simulink model "rfsoc_sdfec_model"  (R2020b)
settings: Solver=VariableStepAuto  StartTime=0.0  StopTime=T  RelTol=1e-3
values from neighbouring files (symbols this model uses):
  aximm_bit_count_reset = 0    [setup.m]
  aximm_bits = n_blocks * k    (= 80)    [setup.m]
  aximm_ctrl_word_dec = 0    [setup.m]
  aximm_ctrl_word_enc = 999    [setup.m]
  aximm_enable = 1    [setup.m]
  aximm_length = k * n_blocks    (= 80)    [setup.m]
  aximm_length_dec = n    (= 160)    [setup.m]
  aximm_length_enc = k/8    (= 10)    [setup.m]
  aximm_llr_scale = (1/noise_var) * llr_scale * 2    (= 200)    [setup.m]
  aximm_noise_std = sqrt(noise_var/2)    [setup.m]
  aximm_reset = 0    [setup.m]
  d = sqrt(-2*log([0:1/4095:1]))    [setup.m]
  fs = 100e6    (= 100000000)    [setup.m]
  generator_polynomial = '''z^13 + z^12 + z^11 + z^8 + 1'''    [setup.m]
libraries: hdlsllib x52, commseqgen3 x28, commblkcod2 x2, simulink x2
(part 2 of 2)

== system rfsoc_sdfec_model/Soft Demodulation/symmetric saturation1 ==
  soft_bits : Inport
  Bit Concat : hdlsllib/Logic and Bit Operations/Bit Concat  numInputs=3
  Bit Slice : hdlsllib/Logic and Bit Operations/Bit Slice  lidx=5  ridx=5
      settings: SourceProductBaseCode=SL
  Constant : Constant  Value=7.75  OutDataTypeStr=fixdt(1,6,2)  SampleTime=-1
  Constant2 : Constant  Value=-7.75  OutDataTypeStr=fixdt(1,6,2)  SampleTime=-1
  GreaterThan : RelationalOperator  Operator=>  OutDataTypeStr=boolean  RndMeth=Simplest
  GreaterThan1 : RelationalOperator  Operator=<  OutDataTypeStr=boolean  RndMeth=Simplest
  Multiport Switch : MultiPortSwitch  DataPortOrder=Zero-based contiguous  Inputs=2  zeroidx=on
  Multiport Switch1 : MultiPortSwitch  DataPortOrder=Zero-based contiguous  Inputs=2  zeroidx=on
  u : Outport
  wires:
  Constant2/1 -> Multiport Switch1/3, GreaterThan1/2
  Constant/1 -> Multiport Switch/3, GreaterThan/2
  Multiport Switch/1 -> Multiport Switch1/2
  GreaterThan1/1 -> Multiport Switch1/1
  GreaterThan/1 -> Multiport Switch/1
  soft_bits/1 -> GreaterThan1/1, Multiport Switch/2, GreaterThan/1
  Bit Concat/1 -> u/1
  Multiport Switch1/1 -> Bit Slice/1, Bit Concat/3
  Bit Slice/1 -> Bit Concat/2, Bit Concat/1

== system rfsoc_sdfec_model/Soft Demodulation/symmetric saturation2 ==
  soft_bits : Inport
  Bit Concat : hdlsllib/Logic and Bit Operations/Bit Concat  numInputs=3
  Bit Slice : hdlsllib/Logic and Bit Operations/Bit Slice  lidx=5  ridx=5
      settings: SourceProductBaseCode=SL
  Constant : Constant  Value=7.75  OutDataTypeStr=fixdt(1,6,2)  SampleTime=-1
  Constant2 : Constant  Value=-7.75  OutDataTypeStr=fixdt(1,6,2)  SampleTime=-1
  GreaterThan : RelationalOperator  Operator=>  OutDataTypeStr=boolean  RndMeth=Simplest
  GreaterThan1 : RelationalOperator  Operator=<  OutDataTypeStr=boolean  RndMeth=Simplest
  Multiport Switch : MultiPortSwitch  DataPortOrder=Zero-based contiguous  Inputs=2  zeroidx=on
  Multiport Switch1 : MultiPortSwitch  DataPortOrder=Zero-based contiguous  Inputs=2  zeroidx=on
  u : Outport
  wires:
  Bit Slice/1 -> Bit Concat/1, Bit Concat/2
  Multiport Switch1/1 -> Bit Concat/3, Bit Slice/1
  Bit Concat/1 -> u/1
  soft_bits/1 -> GreaterThan/1, Multiport Switch/2, GreaterThan1/1
  GreaterThan/1 -> Multiport Switch/1
  GreaterThan1/1 -> Multiport Switch1/1
  Multiport Switch/1 -> Multiport Switch1/2
  Constant/1 -> GreaterThan/2, Multiport Switch/3
  Constant2/1 -> GreaterThan1/2, Multiport Switch1/3

== system rfsoc_sdfec_model/Soft Demodulation/symmetric saturation3 ==
  soft_bits : Inport
  Bit Concat : hdlsllib/Logic and Bit Operations/Bit Concat  numInputs=3
  Bit Slice : hdlsllib/Logic and Bit Operations/Bit Slice  lidx=5  ridx=5
      settings: SourceProductBaseCode=SL
  Constant : Constant  Value=7.75  OutDataTypeStr=fixdt(1,6,2)  SampleTime=-1
  Constant2 : Constant  Value=-7.75  OutDataTypeStr=fixdt(1,6,2)  SampleTime=-1
  GreaterThan : RelationalOperator  Operator=>  OutDataTypeStr=boolean  RndMeth=Simplest
  GreaterThan1 : RelationalOperator  Operator=<  OutDataTypeStr=boolean  RndMeth=Simplest
  Multiport Switch : MultiPortSwitch  DataPortOrder=Zero-based contiguous  Inputs=2  zeroidx=on
  Multiport Switch1 : MultiPortSwitch  DataPortOrder=Zero-based contiguous  Inputs=2  zeroidx=on
  u : Outport
  wires:
  Constant2/1 -> Multiport Switch1/3, GreaterThan1/2
  Constant/1 -> Multiport Switch/3, GreaterThan/2
  Multiport Switch/1 -> Multiport Switch1/2
  GreaterThan1/1 -> Multiport Switch1/1
  GreaterThan/1 -> Multiport Switch/1
  soft_bits/1 -> GreaterThan1/1, Multiport Switch/2, GreaterThan/1
  Bit Concat/1 -> u/1
  Multiport Switch1/1 -> Bit Slice/1, Bit Concat/3
  Bit Slice/1 -> Bit Concat/2, Bit Concat/1

== system rfsoc_sdfec_model/AWGN Channel/AWGN Generator/Random Number Generator ==
  reset : Inport
  enable : EnablePort
  bit0 : commseqgen3/PN Sequence Generator  poly='z^13 + z^12 + z^11 + z^8 + 1'  ini_sta=[ 1 1 1 1 1 1 0 0 1 0 0 0 0]  outBitMaskSource=Dialog parameter  shift=0  outVarSiz=off  maxOutSizeMode=Dialog parameter  maxOutSize=[10 1]  Ts=-1  sampPerFrame=1  reset=on  bitPackedOutputs=off  outDataType=boolean  numPackedBits=8  bitPackDataSigned=off  bitPackedOutDType=double
  bit1 : commseqgen3/PN Sequence Generator  poly='z^13 + z^12 + z^11 + z^8 + 1'  ini_sta=[ 1 1 1 1 1 1 0 0 0 1 0 1 1]  outBitMaskSource=Dialog parameter  shift=0  outVarSiz=off  maxOutSizeMode=Dialog parameter  maxOutSize=[10 1]  Ts=-1  sampPerFrame=1  reset=on  bitPackedOutputs=off  outDataType=boolean  numPackedBits=8  bitPackDataSigned=off  bitPackedOutDType=double
  bit2 : commseqgen3/PN Sequence Generator  poly='z^13 + z^12 + z^11 + z^8 + 1'  ini_sta=[ 0 1 1 1 0 1 0 0 1 1 0 0 0]  outBitMaskSource=Dialog parameter  shift=0  outVarSiz=off  maxOutSizeMode=Dialog parameter  maxOutSize=[10 1]  Ts=-1  sampPerFrame=1  reset=on  bitPackedOutputs=off  outDataType=boolean  numPackedBits=8  bitPackDataSigned=off  bitPackedOutDType=double
  bit3 : commseqgen3/PN Sequence Generator  poly='z^13 + z^12 + z^11 + z^8 + 1'  ini_sta=[ 0 1 0 1 1 0 0 1 0 0 0 1 1]  outBitMaskSource=Dialog parameter  shift=0  outVarSiz=off  maxOutSizeMode=Dialog parameter  maxOutSize=[10 1]  Ts=-1  sampPerFrame=1  reset=on  bitPackedOutputs=off  outDataType=boolean  numPackedBits=8  bitPackDataSigned=off  bitPackedOutDType=double
  bit4 : commseqgen3/PN Sequence Generator  poly='z^13 + z^12 + z^11 + z^8 + 1'  ini_sta=[ 1 1 1 1 1 0 1 1 1 0 1 0 0]  outBitMaskSource=Dialog parameter  shift=0  outVarSiz=off  maxOutSizeMode=Dialog parameter  maxOutSize=[10 1]  Ts=-1  sampPerFrame=1  reset=on  bitPackedOutputs=off  outDataType=boolean  numPackedBits=8  bitPackDataSigned=off  bitPackedOutDType=double
  bit5 : commseqgen3/PN Sequence Generator  poly='z^13 + z^12 + z^11 + z^8 + 1'  ini_sta=[ 0 1 1 1 1 1 0 0 0 1 1 0 0]  outBitMaskSource=Dialog parameter  shift=0  outVarSiz=off  maxOutSizeMode=Dialog parameter  maxOutSize=[10 1]  Ts=-1  sampPerFrame=1  reset=on  bitPackedOutputs=off  outDataType=boolean  numPackedBits=8  bitPackDataSigned=off  bitPackedOutDType=double
  bit6 : commseqgen3/PN Sequence Generator  poly='z^13 + z^12 + z^11 + z^8 + 1'  ini_sta=[ 0 1 0 1 0 0 0 0 1 0 1 0 1]  outBitMaskSource=Dialog parameter  shift=0  outVarSiz=off  maxOutSizeMode=Dialog parameter  maxOutSize=[10 1]  Ts=-1  sampPerFrame=1  reset=on  bitPackedOutputs=off  outDataType=boolean  numPackedBits=8  bitPackDataSigned=off  bitPackedOutDType=double
  bit7 : commseqgen3/PN Sequence Generator  poly='z^13 + z^12 + z^11 + z^8 + 1'  ini_sta=[ 0 1 1 0 0 0 0 1 1 0 1 0 0]  outBitMaskSource=Dialog parameter  shift=0  outVarSiz=off  maxOutSizeMode=Dialog parameter  maxOutSize=[10 1]  Ts=-1  sampPerFrame=1  reset=on  bitPackedOutputs=off  outDataType=boolean  numPackedBits=8  bitPackDataSigned=off  bitPackedOutDType=double
  concat : hdlsllib/Logic and Bit Operations/Bit Concat  numInputs=8
  data : Outport  InitialOutput=0
  wires:
  reset/1 -> bit0/1, bit1/1, bit2/1, bit3/1, bit4/1, bit5/1, bit6/1, bit7/1
  bit0/1 -> concat/1
  bit1/1 -> concat/2
  bit2/1 -> concat/3
  bit3/1 -> concat/4
  bit4/1 -> concat/5
  bit5/1 -> concat/6
  bit6/1 -> concat/7
  bit7/1 -> concat/8
  concat/1 -> data/1

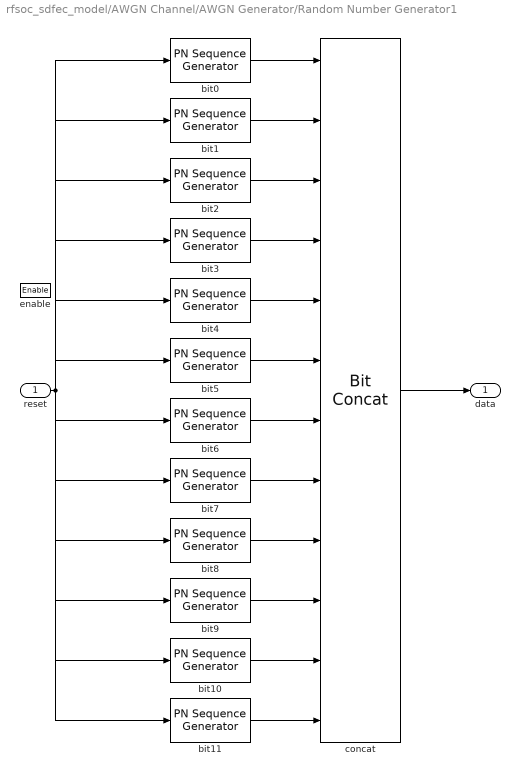
== system rfsoc_sdfec_model/AWGN Channel/AWGN Generator/Random Number Generator1 ==
  reset : Inport
  enable : EnablePort
  bit0 : commseqgen3/PN Sequence Generator  poly='z^13 + z^12 + z^11 + z^8 + 1'  ini_sta=[ 0 1 0 0 0 1 0 1 1 1 0 1 1]  outBitMaskSource=Dialog parameter  shift=0  outVarSiz=off  maxOutSizeMode=Dialog parameter  maxOutSize=[10 1]  Ts=-1  sampPerFrame=1  reset=on  bitPackedOutputs=off  outDataType=boolean  numPackedBits=8  bitPackDataSigned=off  bitPackedOutDType=double
  bit1 : commseqgen3/PN Sequence Generator  poly='z^13 + z^12 + z^11 + z^8 + 1'  ini_sta=[ 1 0 1 0 1 1 0 1 1 0 0 0 1]  outBitMaskSource=Dialog parameter  shift=0  outVarSiz=off  maxOutSizeMode=Dialog parameter  maxOutSize=[10 1]  Ts=-1  sampPerFrame=1  reset=on  bitPackedOutputs=off  outDataType=boolean  numPackedBits=8  bitPackDataSigned=off  bitPackedOutDType=double
  bit10 : commseqgen3/PN Sequence Generator  poly='z^13 + z^12 + z^11 + z^8 + 1'  ini_sta=[ 0 1 1 0 1 1 1 1 1 0 1 0 0]  outBitMaskSource=Dialog parameter  shift=0  outVarSiz=off  maxOutSizeMode=Dialog parameter  maxOutSize=[10 1]  Ts=-1  sampPerFrame=1  reset=on  bitPackedOutputs=off  outDataType=boolean  numPackedBits=8  bitPackDataSigned=off  bitPackedOutDType=double
  bit11 : commseqgen3/PN Sequence Generator  poly='z^13 + z^12 + z^11 + z^8 + 1'  ini_sta=[ 1 1 0 0 1 1 1 1 0 1 1 0 0]  outBitMaskSource=Dialog parameter  shift=0  outVarSiz=off  maxOutSizeMode=Dialog parameter  maxOutSize=[10 1]  Ts=-1  sampPerFrame=1  reset=on  bitPackedOutputs=off  outDataType=boolean  numPackedBits=8  bitPackDataSigned=off  bitPackedOutDType=double
  bit2 : commseqgen3/PN Sequence Generator  poly='z^13 + z^12 + z^11 + z^8 + 1'  ini_sta=[ 0 1 1 1 0 0 1 0 1 0 0 1 1]  outBitMaskSource=Dialog parameter  shift=0  outVarSiz=off  maxOutSizeMode=Dialog parameter  maxOutSize=[10 1]  Ts=-1  sampPerFrame=1  reset=on  bitPackedOutputs=off  outDataType=boolean  numPackedBits=8  bitPackDataSigned=off  bitPackedOutDType=double
  bit3 : commseqgen3/PN Sequence Generator  poly='z^13 + z^12 + z^11 + z^8 + 1'  ini_sta=[ 1 1 1 0 0 1 0 1 1 0 1 1 0]  outBitMaskSource=Dialog parameter  shift=0  outVarSiz=off  maxOutSizeMode=Dialog parameter  maxOutSize=[10 1]  Ts=-1  sampPerFrame=1  reset=on  bitPackedOutputs=off  outDataType=boolean  numPackedBits=8  bitPackDataSigned=off  bitPackedOutDType=double
  bit4 : commseqgen3/PN Sequence Generator  poly='z^13 + z^12 + z^11 + z^8 + 1'  ini_sta=[ 0 1 0 0 1 0 0 0 1 0 1 0 0]  outBitMaskSource=Dialog parameter  shift=0  outVarSiz=off  maxOutSizeMode=Dialog parameter  maxOutSize=[10 1]  Ts=-1  sampPerFrame=1  reset=on  bitPackedOutputs=off  outDataType=boolean  numPackedBits=8  bitPackDataSigned=off  bitPackedOutDType=double
  bit5 : commseqgen3/PN Sequence Generator  poly='z^13 + z^12 + z^11 + z^8 + 1'  ini_sta=[ 1 0 0 0 1 1 1 0 1 1 0 1 1]  outBitMaskSource=Dialog parameter  shift=0  outVarSiz=off  maxOutSizeMode=Dialog parameter  maxOutSize=[10 1]  Ts=-1  sampPerFrame=1  reset=on  bitPackedOutputs=off  outDataType=boolean  numPackedBits=8  bitPackDataSigned=off  bitPackedOutDType=double
  bit6 : commseqgen3/PN Sequence Generator  poly='z^13 + z^12 + z^11 + z^8 + 1'  ini_sta=[ 0 1 0 0 1 1 0 0 0 1 0 0 0]  outBitMaskSource=Dialog parameter  shift=0  outVarSiz=off  maxOutSizeMode=Dialog parameter  maxOutSize=[10 1]  Ts=-1  sampPerFrame=1  reset=on  bitPackedOutputs=off  outDataType=boolean  numPackedBits=8  bitPackDataSigned=off  bitPackedOutDType=double
  bit7 : commseqgen3/PN Sequence Generator  poly='z^13 + z^12 + z^11 + z^8 + 1'  ini_sta=[ 1 1 1 1 0 0 0 1 1 1 1 0 1]  outBitMaskSource=Dialog parameter  shift=0  outVarSiz=off  maxOutSizeMode=Dialog parameter  maxOutSize=[10 1]  Ts=-1  sampPerFrame=1  reset=on  bitPackedOutputs=off  outDataType=boolean  numPackedBits=8  bitPackDataSigned=off  bitPackedOutDType=double
  bit8 : commseqgen3/PN Sequence Generator  poly='z^13 + z^12 + z^11 + z^8 + 1'  ini_sta=[ 1 1 0 0 0 0 0 1 1 0 0 1 1]  outBitMaskSource=Dialog parameter  shift=0  outVarSiz=off  maxOutSizeMode=Dialog parameter  maxOutSize=[10 1]  Ts=-1  sampPerFrame=1  reset=on  bitPackedOutputs=off  outDataType=boolean  numPackedBits=8  bitPackDataSigned=off  bitPackedOutDType=double
  bit9 : commseqgen3/PN Sequence Generator  poly='z^13 + z^12 + z^11 + z^8 + 1'  ini_sta=[ 1 0 0 1 0 0 1 1 0 1 1 1 1]  outBitMaskSource=Dialog parameter  shift=0  outVarSiz=off  maxOutSizeMode=Dialog parameter  maxOutSize=[10 1]  Ts=-1  sampPerFrame=1  reset=on  bitPackedOutputs=off  outDataType=boolean  numPackedBits=8  bitPackDataSigned=off  bitPackedOutDType=double
  concat : hdlsllib/Logic and Bit Operations/Bit Concat  numInputs=12
  data : Outport  InitialOutput=0
  wires:
  reset/1 -> bit0/1, bit1/1, bit2/1, bit3/1, bit4/1, bit5/1, bit6/1, bit7/1, bit8/1, bit9/1, bit10/1, bit11/1
  bit0/1 -> concat/1
  bit1/1 -> concat/2
  bit2/1 -> concat/3
  bit3/1 -> concat/4
  bit4/1 -> concat/5
  bit5/1 -> concat/6
  bit6/1 -> concat/7
  bit7/1 -> concat/8
  bit8/1 -> concat/9
  bit9/1 -> concat/10
  bit10/1 -> concat/11
  bit11/1 -> concat/12
  concat/1 -> data/1

== matlab function rfsoc_sdfec_model/Encoder/MATLAB Function4 ==
  data: bits input; valid input; frame input size=[160, 1]; tvalid output; lane_0 output size=[1,1]
function [tvalid,lane_0] = fcn(bits, valid, frame)

persistent n buffer w buf_i prev_buffer b 

if isempty(n)
    n = 160;
    w = 8;
    b = 0;
    prev_buffer = false(1,w*8*4)';
    buffer = false(1,w*8*4)';
    buf_i = 1;
    lane_0 = uint8(0);
end

coder.extrinsic('binaryVectorToDecimal'); 

tvalid = false;
lane_0(:) = binaryVectorToDecimal(prev_buffer(1:8)','LSBFirst');

if valid
    buffer(buf_i:buf_i + n - 1) = frame;
    buf_i = buf_i + n;
    b = b + 160;
end

if ((b > 0) || (buf_i >= w))
       
    tvalid = true;
    lane_0(:) = binaryVectorToDecimal(buffer(1:8)','LSBFirst');
    b = b - w;
    prev_buffer = buffer;
    
    temp = buffer(w+1:buf_i);
    buf_i = buf_i - w;
    buffer = false(1,w*8*4)';
    buffer(1:buf_i) = temp;
end

== matlab function rfsoc_sdfec_model/Encoder/MATLAB Function3 ==
  data: valid_out output; bits input; valid input; lane_0 input; frame_out output size=[80,1] [80..80]
function [valid_out, frame_out] = fcn(bits, valid, lane_0)

persistent frame fixed_frame frame_i fixed_i k w out_flag bit_count

if isempty(frame)
    k = 80;
    w = 8;
    frame = zeros(1,k)';
    fixed_frame = zeros(1,w*32)';
    frame_i = 1;
    fixed_i = 1;
    out_flag = false;
    bit_count = 0;
end

coder.extrinsic('decimalToBinaryVector');

if valid
    fixed_frame(fixed_i:fixed_i+w) = fliplr(decimalToBinaryVector(lane_0,w));
    fixed_i = fixed_i + w;
end

if fixed_i >= k
    out_flag = true;
end

valid_out = out_flag;

if out_flag
    frame = fixed_frame(frame_i:frame_i+(k-1));
    bit_count = bit_count + k;
    frame_i = frame_i + k;
    if (frame_i + k - 1) > fixed_i - 1
        out_flag = false;
        buf = fixed_frame(frame_i:fixed_i - 1);
        fixed_frame = zeros(1,w*32)';
        fixed_i = fixed_i-frame_i;
        frame_i = 1;
        fixed_frame(1:fixed_i) = buf;
        fixed_i = fixed_i + 1;
    end
end

if (bit_count > bits)
    valid_out = false;
end

frame_out = frame(1:80);

== matlab function rfsoc_sdfec_model/Decode/MATLAB Function5 ==
  data: bits input; valid input; frame input size=[80, 1]; tvalid output; lane_0 output uint8 size=[1,1]
function [tvalid,lane_0] = fcn(bits, valid, frame)

persistent k buffer w buf_i prev_buffer b 

if isempty(k)
    k = 80;
    w = 8;
    prev_buffer = zeros(1,w*8*2)';
    buffer = zeros(1,w*8*2)';
    buf_i = 1;
    lane_0 = uint8(0);
    b = 0;
end

coder.extrinsic('binaryVectorToDecimal'); 

tvalid = false;
lane_0 = uint8(binaryVectorToDecimal(prev_buffer(1:w)','LSBFirst'));

if valid
    buffer(buf_i:buf_i + k - 1) = frame;
    buf_i = buf_i + k;
end

if buf_i >= bits || buf_i >= w
    tvalid = true;
    lane_0 = uint8(binaryVectorToDecimal(buffer(1:w)','LSBFirst'));
    b = b + w;
    
    prev_buffer = buffer;
    
    temp = buffer(w+1:buf_i);
    buf_i = buf_i - w;
    buffer = zeros(1,w*8*2)';
    buffer(1:buf_i) = temp;
    
    if buf_i < 0
        buf_i = 1;
        b = 0;
    end
end

== matlab function rfsoc_sdfec_model/Decode/MATLAB Function1 ==
  data: valid_out output; valid input; lane_0 input; frame_out output size=[160,1] [80..80]
function [valid_out, frame_out] = fcn(valid, lane_0)

persistent frame fixed_frame fixed_i n w

if isempty(frame)
    n = 160;
    w = 32;
    frame = zeros(1,n)';
    fixed_frame = zeros(1,w*32)';
    fixed_i = 1;
end

nt = numerictype(1,6,2);
coder.extrinsic('binaryVectorToDecimal'); 
coder.extrinsic('decimalToBinaryVector');

valid_out = false;

if valid
    lane0_binary = (decimalToBinaryVector(lane_0,w));
    v_0 = binaryVectorToDecimal(lane0_binary(3:8));
    v_0 = reinterpretcast(fi(v_0,0,6,0),nt);
    v_1 = binaryVectorToDecimal(lane0_binary(11:16));
    v_1 = reinterpretcast(fi(v_1,0,6,0),nt);
    v_2 = binaryVectorToDecimal(lane0_binary(19:24));
    v_2 = reinterpretcast(fi(v_2,0,6,0),nt);
    v_3 = binaryVectorToDecimal(lane0_binary(27:32));
    v_3 = reinterpretcast(fi(v_3,0,6,0),nt);
    fixed_frame(fixed_i:fixed_i+3) = [v_0 v_1 v_2 v_3];
    fixed_i = fixed_i + 4;
end

if fixed_i >= n
    frame = fixed_frame(1:160);
    valid_out = true;
    fixed_i = 1;
end

frame_out = frame(1:160);

== matlab function rfsoc_sdfec_model/Soft Demodulation/imag ==
  data: b1 output; b0 output; u input
function [b1, b0] = fcn(u)

if u < -2
    b1 = fi(-2*(u+1),1,16,11);
elseif u > -2 && u < 2
    b1 = fi(-u,1,16,11);
else
    b1 = fi(-2*(u-1),1,16,11);
end

% if u <= 0
%     b0 = fi(u+2,1,16,11);
% else
%     b0 = fi(-u+2,1,16,11);
% end

b0 = fi(-abs(u)+2,1,16,11);

== matlab function rfsoc_sdfec_model/Soft Demodulation/real ==
  data: b3 output; b2 output; u input
function [b3, b2] = fcn(u)

if u < -2
    b3 = fi(2*(u+1),1,16,11);
elseif u >= -2 && u < 2
    b3 = fi(u,1,16,11);
else
    b3 = fi(2*(u-1),1,16,11);
end

b2 = fi(-abs(u)+2,1,16,11);
